simulink model "transition_action"  (R2018b)
settings: Solver=FixedStepDiscrete  StartTime=0.0  StopTime=10.0  RelTol=1e-3
libraries: simulink x1
settings Model: Creator=marwan  LastModifiedBy=marwan

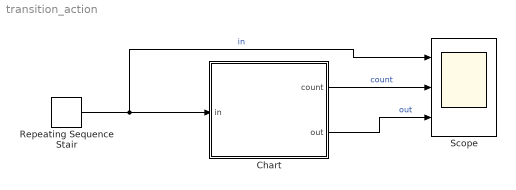
== system transition_action ==
  Chart : Stateflow chart  TreatAsAtomicUnit=on
  Repeating Sequence Stair : simulink/Sources/Repeating Sequence Stair  OutValues=[0 1 1 1 1 1 0 6 6 6]  tsamp=-1  OutMin=[]  OutMax=[]  OutDataTypeStr=double  OutputDataTypeScalingMode=double  OutDataType=fixdt(0,8)  ConRadixGroup=Best Precision: Vector-wise  OutScaling=2^-12
  Scope : Scope  NumInputPorts=3
  wires:
  Chart/1(count) -> Scope/2  "count"
  Chart/2(out) -> Scope/3  "out"
  Repeating Sequence Stair/1 -> Scope/1, Chart/1(in)  "in"

== stateflow chart transition_action/Chart ==
  note: Transition Action:
      | - identified with the mark /
      | - activates oly when the transition from state A to state B is done
      |
      | State Action:
      | - activates only when entering the state
      |
      | Condition Action:
      | - activates only when the condition is TRUE, regardless of the transition has been made or not
  state Out_State
    during:
    count=count-1;
    out=2;
  state Default
    en:
    count=0;
    out=0;
  (default) -> Default
  Default -> (junction 7) : [in>0]{count=count+1;}/{out=1;}
  (junction 7) -> Out_State : [count>3]
  Out_State -> Default : [count<0]
  data: in input; count output; out output
